simulink model "SecRwLtStLgrstInwdOtwdTrgtPosSelc"  (R2018b)
settings: Solver=FixedStepDiscrete  StartTime=0.0  StopTime=10.0  FixedStep=0.01  RelTol=1e-3
undefined symbols (not defined in the file or in its folder): KeSMSw4SAcsMd22SecRwLtStLegrstOtwdInwdPos_Val, KeSMSw4SAcsMd22SecRwLtStLegrstOtwdInwdPosMax_Val, KeSMSw4SAcsMd22SecRwLtStLegrstOtwdInwdPosMin_Val, KeSMSw4SAcsMd26SecRwLtStLegrstOtwdInwdPos_Val, KeSMSw4SAcsMd26SecRwLtStLegrstOtwdInwdPosMax_Val, KeSMSw4SAcsMd26SecRwLtStLegrstOtwdInwdPosMin_Val, KeSMSw4SLegrstCloseMdSecRwLtStLgrstOtwdInwdPos_Val, KeSMSw4SLegrstCloseMdSecRwLtStLgrstOtwdInwdPosMax_Val, KeSMSw4SLegrstCloseMdSecRwLtStLgrstOtwdInwdPosMin_Val, KeSMSw4SLegrstOpenMdSecRwLtStLgrstOtwdInwdPos_Val, KeSMSw4SLegrstOpenMdSecRwLtStLgrstOtwdInwdPosMax_Val, KeSMSw4SLegrstOpenMdSecRwLtStLgrstOtwdInwdPosMin_Val, KeSMSw4sLyingMDSecRwLtStLgrstOtwdInwdPos_160_Val, KeSMSw4sLyingMDSecRwLtStLgrstOtwdInwdPos_165_Val, KeSMSw4sLyingMDSecRwLtStLgrstOtwdInwdPos_170_Val, KeSMSw4sLyingMDSecRwLtStLgrstOtwdInwdPos_175_Val, KeSMSw4sLyingMDSecRwLtStLgrstOtwdInwdPos_180_Val, KeSMSw4sLyingMDSecRwLtStLgrstOtwdInwdPos_Below160_Val, KeSMSw4sLyingMDSecRwLtStLgrstOtwdInwdPos_Over180_Val, KeSMSw4sLyingMDSecRwLtStLgrstOtwdInwdPosMax_160_Val, KeSMSw4sLyingMDSecRwLtStLgrstOtwdInwdPosMax_165_Val, KeSMSw4sLyingMDSecRwLtStLgrstOtwdInwdPosMax_170_Val, KeSMSw4sLyingMDSecRwLtStLgrstOtwdInwdPosMax_175_Val, KeSMSw4sLyingMDSecRwLtStLgrstOtwdInwdPosMax_180_Val, KeSMSw4sLyingMDSecRwLtStLgrstOtwdInwdPosMax_Below160_Val, KeSMSw4sLyingMDSecRwLtStLgrstOtwdInwdPosMax_Over180_Val, KeSMSw4sLyingMDSecRwLtStLgrstOtwdInwdPosMin_160_Val, KeSMSw4sLyingMDSecRwLtStLgrstOtwdInwdPosMin_165_Val, KeSMSw4sLyingMDSecRwLtStLgrstOtwdInwdPosMin_170_Val, KeSMSw4sLyingMDSecRwLtStLgrstOtwdInwdPosMin_175_Val, KeSMSw4sLyingMDSecRwLtStLgrstOtwdInwdPosMin_180_Val, KeSMSw4sLyingMDSecRwLtStLgrstOtwdInwdPosMin_Below160_Val, KeSMSw4sLyingMDSecRwLtStLgrstOtwdInwdPosMin_Over180_Val, KeSMSw4sRecoveryMDSecRwLtStLgrstOtwdInwdPos_160_Val, KeSMSw4sRecoveryMDSecRwLtStLgrstOtwdInwdPos_165_Val, KeSMSw4sRecoveryMDSecRwLtStLgrstOtwdInwdPos_170_Val, KeSMSw4sRecoveryMDSecRwLtStLgrstOtwdInwdPos_175_Val, KeSMSw4sRecoveryMDSecRwLtStLgrstOtwdInwdPos_180_Val, KeSMSw4sRecoveryMDSecRwLtStLgrstOtwdInwdPos_Below160_Val, KeSMSw4sRecoveryMDSecRwLtStLgrstOtwdInwdPos_Over180_Val, KeSMSw4sRecoveryMDSecRwLtStLgrstOtwdInwdPosMax_160_Val, KeSMSw4sRecoveryMDSecRwLtStLgrstOtwdInwdPosMax_165_Val, KeSMSw4sRecoveryMDSecRwLtStLgrstOtwdInwdPosMax_170_Val, KeSMSw4sRecoveryMDSecRwLtStLgrstOtwdInwdPosMax_175_Val, KeSMSw4sRecoveryMDSecRwLtStLgrstOtwdInwdPosMax_180_Val, KeSMSw4sRecoveryMDSecRwLtStLgrstOtwdInwdPosMax_Below160_Val, KeSMSw4sRecoveryMDSecRwLtStLgrstOtwdInwdPosMax_Over180_Val, KeSMSw4sRecoveryMDSecRwLtStLgrstOtwdInwdPosMin_160_Val, KeSMSw4sRecoveryMDSecRwLtStLgrstOtwdInwdPosMin_165_Val, KeSMSw4sRecoveryMDSecRwLtStLgrstOtwdInwdPosMin_170_Val, KeSMSw4sRecoveryMDSecRwLtStLgrstOtwdInwdPosMin_175_Val, KeSMSw4sRecoveryMDSecRwLtStLgrstOtwdInwdPosMin_180_Val, KeSMSw4sRecoveryMDSecRwLtStLgrstOtwdInwdPosMin_Below160_Val, KeSMSw4sRecoveryMDSecRwLtStLgrstOtwdInwdPosMin_Over180_Val, KeSMSw4sVIPMDSecRwLtStLgrstOtwdInwdPos_160_Val, KeSMSw4sVIPMDSecRwLtStLgrstOtwdInwdPos_165_Val, KeSMSw4sVIPMDSecRwLtStLgrstOtwdInwdPos_170_Val, KeSMSw4sVIPMDSecRwLtStLgrstOtwdInwdPos_175_Val, KeSMSw4sVIPMDSecRwLtStLgrstOtwdInwdPos_180_Val, KeSMSw4sVIPMDSecRwLtStLgrstOtwdInwdPos_Below160_Val ... (+36)
libraries: TrgtPosSelcLib x12
(part 1 of 2)
settings Model: Creator=sn2xws  LastModifiedBy=sn2xws
settings Model: ModifiedHistory=|
  | 2023.8.1 V2.0.0 CR401790 增加模式21-26
  | 2024.5.6 V3.0.0 557 67座增加腿托延伸
  | 2024.7.8 V3.0.1 557模式流程V1.9
settings DataIOCC: SaveFormat=StructureWithTime
settings OptimizationCC: DefaultParameterBehavior=Inlined  EnhancedBackFolding=on  PassReuseOutputArgsAs=Individual arguments  ZeroExternalMemoryAtStartup=off  ZeroInternalMemoryAtStartup=off  OptimizeBlockOrder=speed  DifferentSizesBufferReuse=on  OptimizationCustomize=off
settings DebuggingCC: ParameterTunabilityLossMsg=error
settings ModelReferenceCC: ModelReferenceNumInstancesAllowed=Single
settings SFSimCC: MATLABDynamicMemAlloc=off
settings RTWCC: SystemTargetFile=autosar.tlc  GenCodeOnly=on  TemplateMakefile=ert_default_tmf  Description=AUTOSAR  GenerateReport=on  IncludeHyperlinkInReport=on  LaunchReport=on  GenerateTraceInfo=on  GenerateTraceReport=on  GenerateTraceReportSl=on  GenerateTraceReportSf=on  GenerateTraceReportEml=on  GenerateCodeMetricsReport=on
settings CodeAppCC: ForceParamTrailComments=on  IgnoreCustomStorageClasses=off  OperatorAnnotations=on  SimulinkDataObjDesc=on  SFDataObjDesc=on  InsertBlockDesc=on
settings STFCustomTargetCC: TargetLangStandard=C99 (ISO)  MultiwordLength=256  ParMdlRefBuildCompliant=on  CompOptLevelCompliant=on  IncludeMdlTerminateFcn=off  CombineOutputUpdateFcns=on  SuppressErrorStatus=on  ERTCustomFileBanners=on  SupportNonFinite=off  SupportComplex=off  SupportContinuousTime=off  SupportNonInlinedSFcns=off  RemoveResetFunc=on  MATLABClassNameForMDSCustomization=Simulink.SoftwareTarget.ERTCustomization  AutosarCompliant=on  UseToolchainInfoCompliant=on  LookupTableObjectStructAxisOrder=2,1,3,4,...  LUTObjectStructOrderEvenSpacing=Size,Table,Breakpoints  SystemTargetFile=autosar.tlc
settings ERTTargetCC: TargetLangStandard=C99 (ISO)  ConcurrentExecutionCompliant=off  IncludeMdlTerminateFcn=off  SuppressErrorStatus=on  SupportNonFinite=off  SupportComplex=off  ModelStepFunctionPrototypeControlCompliant=off  CPPClassGenCompliant=off  AutosarCompliant=on  LookupTableObjectStructAxisOrder=2,1,3,4,...  LUTObjectStructOrderEvenSpacing=Size,Table,Breakpoints  InlinedParameterPlacement=NonHierarchical  ERTCustomFileTemplate=example_file_process.tlc  ERTFilePackagingFormat=Compact

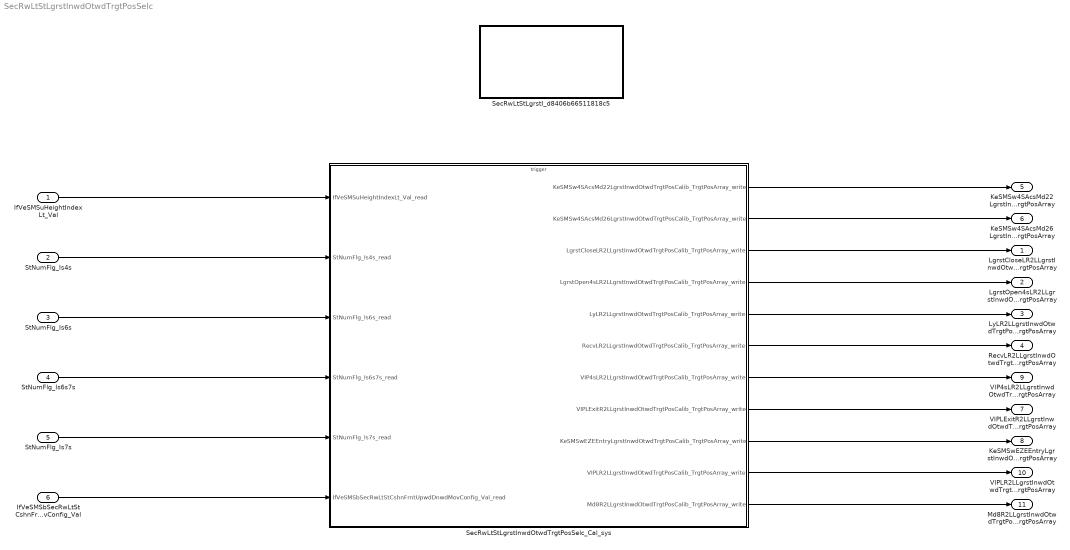
== system SecRwLtStLgrstInwdOtwdTrgtPosSelc ==
  IfVeSMSuHeightIndexLt_Val : Inport  Description=|  OutDataTypeStr=uint8  PortDimensions=1
      | 0：under 160
      | 1：160
      | 2：165
      | 3：170
      | 4：175
      | 5：180
      | 6：over 180
  StNumFlg_Is4s : Inport  Port=2  OutDataTypeStr=boolean  PortDimensions=1
  StNumFlg_Is6s : Inport  Port=3  OutDataTypeStr=boolean  PortDimensions=1
  StNumFlg_Is6s7s : Inport  Port=4  OutDataTypeStr=boolean  PortDimensions=1
  StNumFlg_Is7s : Inport  Port=5  OutDataTypeStr=boolean  PortDimensions=1
  IfVeSMSbSecRwLtStCshnFrntUpwdDnwdMovConfig_Val : Inport  Port=6  OutDataTypeStr=boolean  PortDimensions=1
  SecRwLtStLgrstI_d8406b66511818c5 : Subsystem
  SecRwLtStLgrstInwdOtwdTrgtPosSelc_Cal_sys : Subsystem
  LgrstCloseLR2LLgrstInwdOtwdTrgtPosCalib_TrgtPosArray : Outport  Description=|  OutDataTypeStr=uint16  PortDimensions=3
      | 0:Pos
      | 1:Max
      | 2:Min
  LgrstOpen4sLR2LLgrstInwdOtwdTrgtPosCalib_TrgtPosArray : Outport  Description=|  Port=2  OutDataTypeStr=uint16  PortDimensions=3
      | 0:Pos
      | 1:Max
      | 2:Min
  LyLR2LLgrstInwdOtwdTrgtPosCalib_TrgtPosArray : Outport  Description=|  Port=3  OutDataTypeStr=uint16  PortDimensions=3
      | 0:Pos
      | 1:Max
      | 2:Min
  RecvLR2LLgrstInwdOtwdTrgtPosCalib_TrgtPosArray : Outport  Description=|  Port=4  OutDataTypeStr=uint16  PortDimensions=3
      | 0:Pos
      | 1:Max
      | 2:Min
  KeSMSw4SAcsMd22LgrstInwdOtwdTrgtPosCalib_TrgtPosArray : Outport  Description=|  Port=5  OutDataTypeStr=uint16  PortDimensions=3
      | 0:Pos
      | 1:Max
      | 2:Min
  KeSMSw4SAcsMd26LgrstInwdOtwdTrgtPosCalib_TrgtPosArray : Outport  Description=|  Port=6  OutDataTypeStr=uint16  PortDimensions=3
      | 0:Pos
      | 1:Max
      | 2:Min
  VIPLExitR2LLgrstInwdOtwdTrgtPosCalib_TrgtPosArray : Outport  Description=|  Port=7  OutDataTypeStr=uint16  PortDimensions=3
      | 0:Pos
      | 1:Max
      | 2:Min
  KeSMSwEZEEntryLgrstInwdOtwdTrgtPosCalib_TrgtPosArray : Outport  Description=|  Port=8  OutDataTypeStr=uint16  PortDimensions=3
      | 0:Pos
      | 1:Max
      | 2:Min
  VIP4sLR2LLgrstInwdOtwdTrgtPosCalib_TrgtPosArray : Outport  Description=|  Port=9  OutDataTypeStr=uint16  PortDimensions=3
      | 0:Pos
      | 1:Max
      | 2:Min
  VIPLR2LLgrstInwdOtwdTrgtPosCalib_TrgtPosArray : Outport  Description=|  Port=10  OutDataTypeStr=uint16  PortDimensions=3
      | 0:Pos
      | 1:Max
      | 2:Min
  Md8R2LLgrstInwdOtwdTrgtPosCalib_TrgtPosArray : Outport  Description=|  Port=11  OutDataTypeStr=uint16  PortDimensions=3
      | 0:Pos
      | 1:Max
      | 2:Min
  wires:
  IfVeSMSuHeightIndexLt_Val/1 -> SecRwLtStLgrstInwdOtwdTrgtPosSelc_Cal_sys/1(IfVeSMSuHeightIndexLt_Val_read)
  StNumFlg_Is4s/1 -> SecRwLtStLgrstInwdOtwdTrgtPosSelc_Cal_sys/2(StNumFlg_Is4s_read)
  StNumFlg_Is6s/1 -> SecRwLtStLgrstInwdOtwdTrgtPosSelc_Cal_sys/3(StNumFlg_Is6s_read)
  StNumFlg_Is6s7s/1 -> SecRwLtStLgrstInwdOtwdTrgtPosSelc_Cal_sys/4(StNumFlg_Is6s7s_read)
  StNumFlg_Is7s/1 -> SecRwLtStLgrstInwdOtwdTrgtPosSelc_Cal_sys/5(StNumFlg_Is7s_read)
  SecRwLtStLgrstInwdOtwdTrgtPosSelc_Cal_sys/3(LgrstCloseLR2LLgrstInwdOtwdTrgtPosCalib_TrgtPosArray_write) -> LgrstCloseLR2LLgrstInwdOtwdTrgtPosCalib_TrgtPosArray/1
  SecRwLtStLgrstInwdOtwdTrgtPosSelc_Cal_sys/4(LgrstOpen4sLR2LLgrstInwdOtwdTrgtPosCalib_TrgtPosArray_write) -> LgrstOpen4sLR2LLgrstInwdOtwdTrgtPosCalib_TrgtPosArray/1
  SecRwLtStLgrstInwdOtwdTrgtPosSelc_Cal_sys/5(LyLR2LLgrstInwdOtwdTrgtPosCalib_TrgtPosArray_write) -> LyLR2LLgrstInwdOtwdTrgtPosCalib_TrgtPosArray/1
  SecRwLtStLgrstInwdOtwdTrgtPosSelc_Cal_sys/6(RecvLR2LLgrstInwdOtwdTrgtPosCalib_TrgtPosArray_write) -> RecvLR2LLgrstInwdOtwdTrgtPosCalib_TrgtPosArray/1
  SecRwLtStLgrstInwdOtwdTrgtPosSelc_Cal_sys/1(KeSMSw4SAcsMd22LgrstInwdOtwdTrgtPosCalib_TrgtPosArray_write) -> KeSMSw4SAcsMd22LgrstInwdOtwdTrgtPosCalib_TrgtPosArray/1
  SecRwLtStLgrstInwdOtwdTrgtPosSelc_Cal_sys/2(KeSMSw4SAcsMd26LgrstInwdOtwdTrgtPosCalib_TrgtPosArray_write) -> KeSMSw4SAcsMd26LgrstInwdOtwdTrgtPosCalib_TrgtPosArray/1
  IfVeSMSbSecRwLtStCshnFrntUpwdDnwdMovConfig_Val/1 -> SecRwLtStLgrstInwdOtwdTrgtPosSelc_Cal_sys/6(IfVeSMSbSecRwLtStCshnFrntUpwdDnwdMovConfig_Val_read)
  SecRwLtStLgrstInwdOtwdTrgtPosSelc_Cal_sys/8(VIPLExitR2LLgrstInwdOtwdTrgtPosCalib_TrgtPosArray_write) -> VIPLExitR2LLgrstInwdOtwdTrgtPosCalib_TrgtPosArray/1
  SecRwLtStLgrstInwdOtwdTrgtPosSelc_Cal_sys/9(KeSMSwEZEEntryLgrstInwdOtwdTrgtPosCalib_TrgtPosArray_write) -> KeSMSwEZEEntryLgrstInwdOtwdTrgtPosCalib_TrgtPosArray/1
  SecRwLtStLgrstInwdOtwdTrgtPosSelc_Cal_sys/7(VIP4sLR2LLgrstInwdOtwdTrgtPosCalib_TrgtPosArray_write) -> VIP4sLR2LLgrstInwdOtwdTrgtPosCalib_TrgtPosArray/1
  SecRwLtStLgrstInwdOtwdTrgtPosSelc_Cal_sys/10(VIPLR2LLgrstInwdOtwdTrgtPosCalib_TrgtPosArray_write) -> VIPLR2LLgrstInwdOtwdTrgtPosCalib_TrgtPosArray/1
  SecRwLtStLgrstInwdOtwdTrgtPosSelc_Cal_sys/11(Md8R2LLgrstInwdOtwdTrgtPosCalib_TrgtPosArray_write) -> Md8R2LLgrstInwdOtwdTrgtPosCalib_TrgtPosArray/1

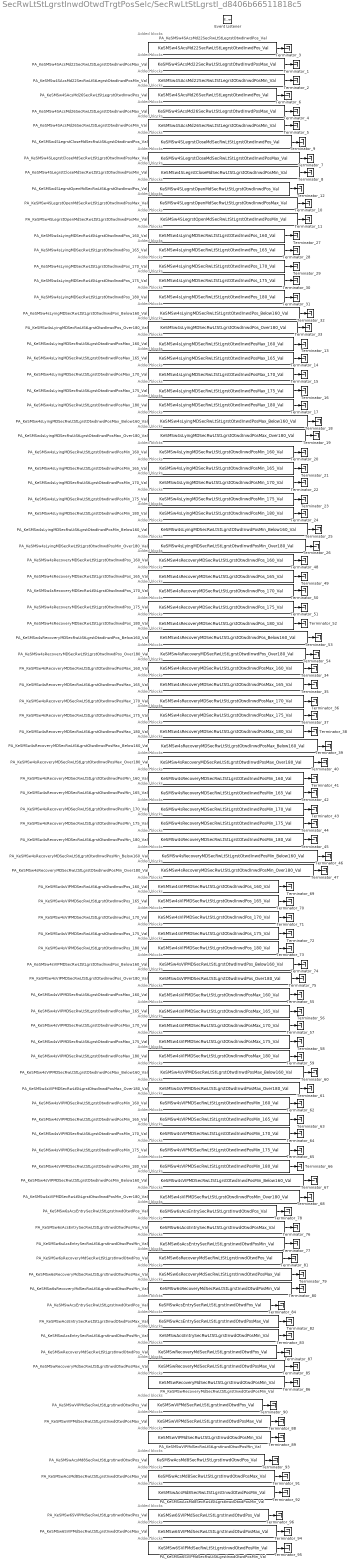
== system SecRwLtStLgrstInwdOtwdTrgtPosSelc/SecRwLtStLgrstI_d8406b66511818c5 ==
  note: Added blocks
  note: Added blocks
  note: Added blocks
  note: Added blocks
  note: Added blocks
  note: Added blocks
  note: Added blocks
  note: Added blocks
  note: Added blocks
  note: Added blocks
  note: Added blocks
  note: Added blocks
  note: Added blocks
  note: Added blocks
  note: Added blocks
  note: Added blocks
  note: Added blocks
  note: Added blocks
  note: Added blocks
  note: Added blocks
  note: Added blocks
  note: Added blocks
  note: Added blocks
  note: Added blocks
  note: Added blocks
  note: Added blocks
  note: Added blocks
  note: Added blocks
  note: Added blocks
  note: Added blocks
  note: Added blocks
  note: Added blocks
  note: Added blocks
  note: Added blocks
  note: Added blocks
  note: Added blocks
  note: Added blocks
  note: Added blocks
  note: Added blocks
  note: Added blocks
  note: Added blocks
  note: Added blocks
  note: Added blocks
  note: Added blocks
  note: Added blocks
  note: Added blocks
  note: Added blocks
  note: Added blocks
  note: Added blocks
  note: Added blocks
  note: Added blocks
  note: Added blocks
  note: Added blocks
  note: Added blocks
  note: Added blocks
  note: Added blocks
  note: Added blocks
  note: Added blocks
  note: Added blocks
  note: Added blocks
  note: Added blocks
  note: Added blocks
  note: Added blocks
  note: Added blocks
  note: Added blocks
  note: Added blocks
  note: Added blocks
  note: Added blocks
  note: Added blocks
  note: Added blocks
  note: Added blocks
  note: Added blocks
  note: Added blocks
  note: Added blocks
  note: Added blocks
  note: Added blocks
  note: Added blocks
  note: Added blocks
  note: Added blocks
  note: Added blocks
  note: Added blocks
  note: Added blocks
  note: Added blocks
  note: Added blocks
  note: Added blocks
  note: Added blocks
  note: Added blocks
  note: Added blocks
  note: Added blocks
  note: Added blocks
  note: Added blocks
  note: Added blocks
  note: Added blocks
  note: Added blocks
  note: Added blocks
  note: Added blocks
  Event Listener : EventListener  EventName=reset
  PA_KeSMSw4SAcsMd22SecRwLtStLegrstOtwdInwdPosMax_Val : Constant  Value=KeSMSw4SAcsMd22SecRwLtStLegrstOtwdInwdPosMax_Val
  PA_KeSMSw4SAcsMd22SecRwLtStLegrstOtwdInwdPosMin_Val : Constant  Value=KeSMSw4SAcsMd22SecRwLtStLegrstOtwdInwdPosMin_Val
  PA_KeSMSw4SAcsMd22SecRwLtStLegrstOtwdInwdPos_Val : Constant  Value=KeSMSw4SAcsMd22SecRwLtStLegrstOtwdInwdPos_Val
  PA_KeSMSw4SAcsMd26SecRwLtStLegrstOtwdInwdPosMax_Val : Constant  Value=KeSMSw4SAcsMd26SecRwLtStLegrstOtwdInwdPosMax_Val
  PA_KeSMSw4SAcsMd26SecRwLtStLegrstOtwdInwdPosMin_Val : Constant  Value=KeSMSw4SAcsMd26SecRwLtStLegrstOtwdInwdPosMin_Val
  PA_KeSMSw4SAcsMd26SecRwLtStLegrstOtwdInwdPos_Val : Constant  Value=KeSMSw4SAcsMd26SecRwLtStLegrstOtwdInwdPos_Val
  PA_KeSMSw4SLegrstCloseMdSecRwLtStLgrstOtwdInwdPosMax_Val : Constant  Value=KeSMSw4SLegrstCloseMdSecRwLtStLgrstOtwdInwdPosMax_Val
  PA_KeSMSw4SLegrstCloseMdSecRwLtStLgrstOtwdInwdPosMin_Val : Constant  Value=KeSMSw4SLegrstCloseMdSecRwLtStLgrstOtwdInwdPosMin_Val
  PA_KeSMSw4SLegrstCloseMdSecRwLtStLgrstOtwdInwdPos_Val : Constant  Value=KeSMSw4SLegrstCloseMdSecRwLtStLgrstOtwdInwdPos_Val
  PA_KeSMSw4SLegrstOpenMdSecRwLtStLgrstOtwdInwdPosMax_Val : Constant  Value=KeSMSw4SLegrstOpenMdSecRwLtStLgrstOtwdInwdPosMax_Val
  PA_KeSMSw4SLegrstOpenMdSecRwLtStLgrstOtwdInwdPosMin_Val : Constant  Value=KeSMSw4SLegrstOpenMdSecRwLtStLgrstOtwdInwdPosMin_Val
  PA_KeSMSw4SLegrstOpenMdSecRwLtStLgrstOtwdInwdPos_Val : Constant  Value=KeSMSw4SLegrstOpenMdSecRwLtStLgrstOtwdInwdPos_Val
  PA_KeSMSw4sLyingMDSecRwLtStLgrstOtwdInwdPosMax_160_Val : Constant  Value=KeSMSw4sLyingMDSecRwLtStLgrstOtwdInwdPosMax_160_Val
  PA_KeSMSw4sLyingMDSecRwLtStLgrstOtwdInwdPosMax_165_Val : Constant  Value=KeSMSw4sLyingMDSecRwLtStLgrstOtwdInwdPosMax_165_Val
  PA_KeSMSw4sLyingMDSecRwLtStLgrstOtwdInwdPosMax_170_Val : Constant  Value=KeSMSw4sLyingMDSecRwLtStLgrstOtwdInwdPosMax_170_Val
  PA_KeSMSw4sLyingMDSecRwLtStLgrstOtwdInwdPosMax_175_Val : Constant  Value=KeSMSw4sLyingMDSecRwLtStLgrstOtwdInwdPosMax_175_Val
  PA_KeSMSw4sLyingMDSecRwLtStLgrstOtwdInwdPosMax_180_Val : Constant  Value=KeSMSw4sLyingMDSecRwLtStLgrstOtwdInwdPosMax_180_Val
  PA_KeSMSw4sLyingMDSecRwLtStLgrstOtwdInwdPosMax_Below160_Val : Constant  Value=KeSMSw4sLyingMDSecRwLtStLgrstOtwdInwdPosMax_Below160_Val
  PA_KeSMSw4sLyingMDSecRwLtStLgrstOtwdInwdPosMax_Over180_Val : Constant  Value=KeSMSw4sLyingMDSecRwLtStLgrstOtwdInwdPosMax_Over180_Val
  PA_KeSMSw4sLyingMDSecRwLtStLgrstOtwdInwdPosMin_160_Val : Constant  Value=KeSMSw4sLyingMDSecRwLtStLgrstOtwdInwdPosMin_160_Val
  PA_KeSMSw4sLyingMDSecRwLtStLgrstOtwdInwdPosMin_165_Val : Constant  Value=KeSMSw4sLyingMDSecRwLtStLgrstOtwdInwdPosMin_165_Val
  PA_KeSMSw4sLyingMDSecRwLtStLgrstOtwdInwdPosMin_170_Val : Constant  Value=KeSMSw4sLyingMDSecRwLtStLgrstOtwdInwdPosMin_170_Val
  PA_KeSMSw4sLyingMDSecRwLtStLgrstOtwdInwdPosMin_175_Val : Constant  Value=KeSMSw4sLyingMDSecRwLtStLgrstOtwdInwdPosMin_175_Val
  PA_KeSMSw4sLyingMDSecRwLtStLgrstOtwdInwdPosMin_180_Val : Constant  Value=KeSMSw4sLyingMDSecRwLtStLgrstOtwdInwdPosMin_180_Val
  PA_KeSMSw4sLyingMDSecRwLtStLgrstOtwdInwdPosMin_Below160_Val : Constant  Value=KeSMSw4sLyingMDSecRwLtStLgrstOtwdInwdPosMin_Below160_Val
  PA_KeSMSw4sLyingMDSecRwLtStLgrstOtwdInwdPosMin_Over180_Val : Constant  Value=KeSMSw4sLyingMDSecRwLtStLgrstOtwdInwdPosMin_Over180_Val
  PA_KeSMSw4sLyingMDSecRwLtStLgrstOtwdInwdPos_160_Val : Constant  Value=KeSMSw4sLyingMDSecRwLtStLgrstOtwdInwdPos_160_Val
  PA_KeSMSw4sLyingMDSecRwLtStLgrstOtwdInwdPos_165_Val : Constant  Value=KeSMSw4sLyingMDSecRwLtStLgrstOtwdInwdPos_165_Val
  PA_KeSMSw4sLyingMDSecRwLtStLgrstOtwdInwdPos_170_Val : Constant  Value=KeSMSw4sLyingMDSecRwLtStLgrstOtwdInwdPos_170_Val
  PA_KeSMSw4sLyingMDSecRwLtStLgrstOtwdInwdPos_175_Val : Constant  Value=KeSMSw4sLyingMDSecRwLtStLgrstOtwdInwdPos_175_Val
  PA_KeSMSw4sLyingMDSecRwLtStLgrstOtwdInwdPos_180_Val : Constant  Value=KeSMSw4sLyingMDSecRwLtStLgrstOtwdInwdPos_180_Val
  PA_KeSMSw4sLyingMDSecRwLtStLgrstOtwdInwdPos_Below160_Val : Constant  Value=KeSMSw4sLyingMDSecRwLtStLgrstOtwdInwdPos_Below160_Val
  PA_KeSMSw4sLyingMDSecRwLtStLgrstOtwdInwdPos_Over180_Val : Constant  Value=KeSMSw4sLyingMDSecRwLtStLgrstOtwdInwdPos_Over180_Val
  PA_KeSMSw4sRecoveryMDSecRwLtStLgrstOtwdInwdPosMax_160_Val : Constant  Value=KeSMSw4sRecoveryMDSecRwLtStLgrstOtwdInwdPosMax_160_Val
  PA_KeSMSw4sRecoveryMDSecRwLtStLgrstOtwdInwdPosMax_165_Val : Constant  Value=KeSMSw4sRecoveryMDSecRwLtStLgrstOtwdInwdPosMax_165_Val
  PA_KeSMSw4sRecoveryMDSecRwLtStLgrstOtwdInwdPosMax_170_Val : Constant  Value=KeSMSw4sRecoveryMDSecRwLtStLgrstOtwdInwdPosMax_170_Val
  PA_KeSMSw4sRecoveryMDSecRwLtStLgrstOtwdInwdPosMax_175_Val : Constant  Value=KeSMSw4sRecoveryMDSecRwLtStLgrstOtwdInwdPosMax_175_Val
  PA_KeSMSw4sRecoveryMDSecRwLtStLgrstOtwdInwdPosMax_180_Val : Constant  Value=KeSMSw4sRecoveryMDSecRwLtStLgrstOtwdInwdPosMax_180_Val
  PA_KeSMSw4sRecoveryMDSecRwLtStLgrstOtwdInwdPosMax_Below160_Val : Constant  Value=KeSMSw4sRecoveryMDSecRwLtStLgrstOtwdInwdPosMax_Below160_Val
  PA_KeSMSw4sRecoveryMDSecRwLtStLgrstOtwdInwdPosMax_Over180_Val : Constant  Value=KeSMSw4sRecoveryMDSecRwLtStLgrstOtwdInwdPosMax_Over180_Val
  PA_KeSMSw4sRecoveryMDSecRwLtStLgrstOtwdInwdPosMin_160_Val : Constant  Value=KeSMSw4sRecoveryMDSecRwLtStLgrstOtwdInwdPosMin_160_Val
  PA_KeSMSw4sRecoveryMDSecRwLtStLgrstOtwdInwdPosMin_165_Val : Constant  Value=KeSMSw4sRecoveryMDSecRwLtStLgrstOtwdInwdPosMin_165_Val
  PA_KeSMSw4sRecoveryMDSecRwLtStLgrstOtwdInwdPosMin_170_Val : Constant  Value=KeSMSw4sRecoveryMDSecRwLtStLgrstOtwdInwdPosMin_170_Val
  PA_KeSMSw4sRecoveryMDSecRwLtStLgrstOtwdInwdPosMin_175_Val : Constant  Value=KeSMSw4sRecoveryMDSecRwLtStLgrstOtwdInwdPosMin_175_Val
  PA_KeSMSw4sRecoveryMDSecRwLtStLgrstOtwdInwdPosMin_180_Val : Constant  Value=KeSMSw4sRecoveryMDSecRwLtStLgrstOtwdInwdPosMin_180_Val
  PA_KeSMSw4sRecoveryMDSecRwLtStLgrstOtwdInwdPosMin_Below160_Val : Constant  Value=KeSMSw4sRecoveryMDSecRwLtStLgrstOtwdInwdPosMin_Below160_Val
  PA_KeSMSw4sRecoveryMDSecRwLtStLgrstOtwdInwdPosMin_Over180_Val : Constant  Value=KeSMSw4sRecoveryMDSecRwLtStLgrstOtwdInwdPosMin_Over180_Val
  PA_KeSMSw4sRecoveryMDSecRwLtStLgrstOtwdInwdPos_160_Val : Constant  Value=KeSMSw4sRecoveryMDSecRwLtStLgrstOtwdInwdPos_160_Val
  PA_KeSMSw4sRecoveryMDSecRwLtStLgrstOtwdInwdPos_165_Val : Constant  Value=KeSMSw4sRecoveryMDSecRwLtStLgrstOtwdInwdPos_165_Val
  PA_KeSMSw4sRecoveryMDSecRwLtStLgrstOtwdInwdPos_170_Val : Constant  Value=KeSMSw4sRecoveryMDSecRwLtStLgrstOtwdInwdPos_170_Val
  PA_KeSMSw4sRecoveryMDSecRwLtStLgrstOtwdInwdPos_175_Val : Constant  Value=KeSMSw4sRecoveryMDSecRwLtStLgrstOtwdInwdPos_175_Val
  PA_KeSMSw4sRecoveryMDSecRwLtStLgrstOtwdInwdPos_180_Val : Constant  Value=KeSMSw4sRecoveryMDSecRwLtStLgrstOtwdInwdPos_180_Val
  PA_KeSMSw4sRecoveryMDSecRwLtStLgrstOtwdInwdPos_Below160_Val : Constant  Value=KeSMSw4sRecoveryMDSecRwLtStLgrstOtwdInwdPos_Below160_Val
  PA_KeSMSw4sRecoveryMDSecRwLtStLgrstOtwdInwdPos_Over180_Val : Constant  Value=KeSMSw4sRecoveryMDSecRwLtStLgrstOtwdInwdPos_Over180_Val
  PA_KeSMSw4sVIPMDSecRwLtStLgrstOtwdInwdPosMax_160_Val : Constant  Value=KeSMSw4sVIPMDSecRwLtStLgrstOtwdInwdPosMax_160_Val
  PA_KeSMSw4sVIPMDSecRwLtStLgrstOtwdInwdPosMax_165_Val : Constant  Value=KeSMSw4sVIPMDSecRwLtStLgrstOtwdInwdPosMax_165_Val
  PA_KeSMSw4sVIPMDSecRwLtStLgrstOtwdInwdPosMax_170_Val : Constant  Value=KeSMSw4sVIPMDSecRwLtStLgrstOtwdInwdPosMax_170_Val
  PA_KeSMSw4sVIPMDSecRwLtStLgrstOtwdInwdPosMax_175_Val : Constant  Value=KeSMSw4sVIPMDSecRwLtStLgrstOtwdInwdPosMax_175_Val
  PA_KeSMSw4sVIPMDSecRwLtStLgrstOtwdInwdPosMax_180_Val : Constant  Value=KeSMSw4sVIPMDSecRwLtStLgrstOtwdInwdPosMax_180_Val
  PA_KeSMSw4sVIPMDSecRwLtStLgrstOtwdInwdPosMax_Below160_Val : Constant  Value=KeSMSw4sVIPMDSecRwLtStLgrstOtwdInwdPosMax_Below160_Val
  PA_KeSMSw4sVIPMDSecRwLtStLgrstOtwdInwdPosMax_Over180_Val : Constant  Value=KeSMSw4sVIPMDSecRwLtStLgrstOtwdInwdPosMax_Over180_Val
  PA_KeSMSw4sVIPMDSecRwLtStLgrstOtwdInwdPosMin_160_Val : Constant  Value=KeSMSw4sVIPMDSecRwLtStLgrstOtwdInwdPosMin_160_Val
  PA_KeSMSw4sVIPMDSecRwLtStLgrstOtwdInwdPosMin_165_Val : Constant  Value=KeSMSw4sVIPMDSecRwLtStLgrstOtwdInwdPosMin_165_Val
  PA_KeSMSw4sVIPMDSecRwLtStLgrstOtwdInwdPosMin_170_Val : Constant  Value=KeSMSw4sVIPMDSecRwLtStLgrstOtwdInwdPosMin_170_Val
  PA_KeSMSw4sVIPMDSecRwLtStLgrstOtwdInwdPosMin_175_Val : Constant  Value=KeSMSw4sVIPMDSecRwLtStLgrstOtwdInwdPosMin_175_Val
  PA_KeSMSw4sVIPMDSecRwLtStLgrstOtwdInwdPosMin_180_Val : Constant  Value=KeSMSw4sVIPMDSecRwLtStLgrstOtwdInwdPosMin_180_Val
  PA_KeSMSw4sVIPMDSecRwLtStLgrstOtwdInwdPosMin_Below160_Val : Constant  Value=KeSMSw4sVIPMDSecRwLtStLgrstOtwdInwdPosMin_Below160_Val
  PA_KeSMSw4sVIPMDSecRwLtStLgrstOtwdInwdPosMin_Over180_Val : Constant  Value=KeSMSw4sVIPMDSecRwLtStLgrstOtwdInwdPosMin_Over180_Val
  PA_KeSMSw4sVIPMDSecRwLtStLgrstOtwdInwdPos_160_Val : Constant  Value=KeSMSw4sVIPMDSecRwLtStLgrstOtwdInwdPos_160_Val
  PA_KeSMSw4sVIPMDSecRwLtStLgrstOtwdInwdPos_165_Val : Constant  Value=KeSMSw4sVIPMDSecRwLtStLgrstOtwdInwdPos_165_Val
  PA_KeSMSw4sVIPMDSecRwLtStLgrstOtwdInwdPos_170_Val : Constant  Value=KeSMSw4sVIPMDSecRwLtStLgrstOtwdInwdPos_170_Val
  PA_KeSMSw4sVIPMDSecRwLtStLgrstOtwdInwdPos_175_Val : Constant  Value=KeSMSw4sVIPMDSecRwLtStLgrstOtwdInwdPos_175_Val
  PA_KeSMSw4sVIPMDSecRwLtStLgrstOtwdInwdPos_180_Val : Constant  Value=KeSMSw4sVIPMDSecRwLtStLgrstOtwdInwdPos_180_Val
  PA_KeSMSw4sVIPMDSecRwLtStLgrstOtwdInwdPos_Below160_Val : Constant  Value=KeSMSw4sVIPMDSecRwLtStLgrstOtwdInwdPos_Below160_Val
  PA_KeSMSw4sVIPMDSecRwLtStLgrstOtwdInwdPos_Over180_Val : Constant  Value=KeSMSw4sVIPMDSecRwLtStLgrstOtwdInwdPos_Over180_Val
  PA_KeSMSw6SVIPMdSecRwLtStLgrstInwdOtwdPosMax_Val : Constant  Value=KeSMSw6SVIPMdSecRwLtStLgrstInwdOtwdPosMax_Val
  PA_KeSMSw6SVIPMdSecRwLtStLgrstInwdOtwdPosMin_Val : Constant  Value=KeSMSw6SVIPMdSecRwLtStLgrstInwdOtwdPosMin_Val
  PA_KeSMSw6SVIPMdSecRwLtStLgrstInwdOtwdPos_Val : Constant  Value=KeSMSw6SVIPMdSecRwLtStLgrstInwdOtwdPos_Val
  PA_KeSMSw6sAcsEntrySecRwLtStLgrstInwdOtwdPosMax_Val : Constant  Value=KeSMSw6sAcsEntrySecRwLtStLgrstInwdOtwdPosMax_Val
  PA_KeSMSw6sAcsEntrySecRwLtStLgrstInwdOtwdPosMin_Val : Constant  Value=KeSMSw6sAcsEntrySecRwLtStLgrstInwdOtwdPosMin_Val
  PA_KeSMSw6sAcsEntrySecRwLtStLgrstInwdOtwdPos_Val : Constant  Value=KeSMSw6sAcsEntrySecRwLtStLgrstInwdOtwdPos_Val
  PA_KeSMSw6sRecoveryMdSecRwLtStLgrstInwdOtwdPosMax_Val : Constant  Value=KeSMSw6sRecoveryMdSecRwLtStLgrstInwdOtwdPosMax_Val
  PA_KeSMSw6sRecoveryMdSecRwLtStLgrstInwdOtwdPosMin_Val : Constant  Value=KeSMSw6sRecoveryMdSecRwLtStLgrstInwdOtwdPosMin_Val
  PA_KeSMSw6sRecoveryMdSecRwLtStLgrstInwdOtwdPos_Val : Constant  Value=KeSMSw6sRecoveryMdSecRwLtStLgrstInwdOtwdPos_Val
  PA_KeSMSwAcsEntrySecRwLtStLgrstInwdOtwdPosMax_Val : Constant  Value=KeSMSwAcsEntrySecRwLtStLgrstInwdOtwdPosMax_Val
  PA_KeSMSwAcsEntrySecRwLtStLgrstInwdOtwdPosMin_Val : Constant  Value=KeSMSwAcsEntrySecRwLtStLgrstInwdOtwdPosMin_Val
  PA_KeSMSwAcsEntrySecRwLtStLgrstInwdOtwdPos_Val : Constant  Value=KeSMSwAcsEntrySecRwLtStLgrstInwdOtwdPos_Val
  PA_KeSMSwAcsMd8SecRwLtStLgrstInwdOtwdPosMax_Val : Constant  Value=KeSMSwAcsMd8SecRwLtStLgrstInwdOtwdPosMax_Val
  PA_KeSMSwAcsMd8SecRwLtStLgrstInwdOtwdPosMin_Val : Constant  Value=KeSMSwAcsMd8SecRwLtStLgrstInwdOtwdPosMin_Val
  PA_KeSMSwAcsMd8SecRwLtStLgrstInwdOtwdPos_Val : Constant  Value=KeSMSwAcsMd8SecRwLtStLgrstInwdOtwdPos_Val
  PA_KeSMSwRecoveryMdSecRwLtStLgrstInwdOtwdPosMax_Val : Constant  Value=KeSMSwRecoveryMdSecRwLtStLgrstInwdOtwdPosMax_Val
  PA_KeSMSwRecoveryMdSecRwLtStLgrstInwdOtwdPosMin_Val : Constant  Value=KeSMSwRecoveryMdSecRwLtStLgrstInwdOtwdPosMin_Val
  PA_KeSMSwRecoveryMdSecRwLtStLgrstInwdOtwdPos_Val : Constant  Value=KeSMSwRecoveryMdSecRwLtStLgrstInwdOtwdPos_Val
  PA_KeSMSwVIPMdSecRwLtStLgrstInwdOtwdPosMax_Val : Constant  Value=KeSMSwVIPMdSecRwLtStLgrstInwdOtwdPosMax_Val
  PA_KeSMSwVIPMdSecRwLtStLgrstInwdOtwdPosMin_Val : Constant  Value=KeSMSwVIPMdSecRwLtStLgrstInwdOtwdPosMin_Val
  PA_KeSMSwVIPMdSecRwLtStLgrstInwdOtwdPos_Val : Constant  Value=KeSMSwVIPMdSecRwLtStLgrstInwdOtwdPos_Val
  Terminator_{1..96} (96 alike) : Terminator
  wires:
  PA_KeSMSw4SAcsMd22SecRwLtStLegrstOtwdInwdPosMax_Val/1 -> Terminator_1/1
  PA_KeSMSw4SAcsMd22SecRwLtStLegrstOtwdInwdPosMin_Val/1 -> Terminator_2/1
  PA_KeSMSw4SAcsMd22SecRwLtStLegrstOtwdInwdPos_Val/1 -> Terminator_3/1
  PA_KeSMSw4SAcsMd26SecRwLtStLegrstOtwdInwdPosMax_Val/1 -> Terminator_4/1
  PA_KeSMSw4SAcsMd26SecRwLtStLegrstOtwdInwdPosMin_Val/1 -> Terminator_5/1
  PA_KeSMSw4SAcsMd26SecRwLtStLegrstOtwdInwdPos_Val/1 -> Terminator_6/1
  PA_KeSMSw4SLegrstCloseMdSecRwLtStLgrstOtwdInwdPosMax_Val/1 -> Terminator_7/1
  PA_KeSMSw4SLegrstCloseMdSecRwLtStLgrstOtwdInwdPosMin_Val/1 -> Terminator_8/1
  PA_KeSMSw4SLegrstCloseMdSecRwLtStLgrstOtwdInwdPos_Val/1 -> Terminator_9/1
  PA_KeSMSw4SLegrstOpenMdSecRwLtStLgrstOtwdInwdPosMax_Val/1 -> Terminator_10/1
  PA_KeSMSw4SLegrstOpenMdSecRwLtStLgrstOtwdInwdPosMin_Val/1 -> Terminator_11/1
  PA_KeSMSw4SLegrstOpenMdSecRwLtStLgrstOtwdInwdPos_Val/1 -> Terminator_12/1
  PA_KeSMSw4sLyingMDSecRwLtStLgrstOtwdInwdPosMax_160_Val/1 -> Terminator_13/1
  PA_KeSMSw4sLyingMDSecRwLtStLgrstOtwdInwdPosMax_165_Val/1 -> Terminator_14/1
  PA_KeSMSw4sLyingMDSecRwLtStLgrstOtwdInwdPosMax_170_Val/1 -> Terminator_15/1
  PA_KeSMSw4sLyingMDSecRwLtStLgrstOtwdInwdPosMax_175_Val/1 -> Terminator_16/1
  PA_KeSMSw4sLyingMDSecRwLtStLgrstOtwdInwdPosMax_180_Val/1 -> Terminator_17/1
  PA_KeSMSw4sLyingMDSecRwLtStLgrstOtwdInwdPosMax_Below160_Val/1 -> Terminator_18/1
  PA_KeSMSw4sLyingMDSecRwLtStLgrstOtwdInwdPosMax_Over180_Val/1 -> Terminator_19/1
  PA_KeSMSw4sLyingMDSecRwLtStLgrstOtwdInwdPosMin_160_Val/1 -> Terminator_20/1
  PA_KeSMSw4sLyingMDSecRwLtStLgrstOtwdInwdPosMin_165_Val/1 -> Terminator_21/1
  PA_KeSMSw4sLyingMDSecRwLtStLgrstOtwdInwdPosMin_170_Val/1 -> Terminator_22/1
  PA_KeSMSw4sLyingMDSecRwLtStLgrstOtwdInwdPosMin_175_Val/1 -> Terminator_23/1
  PA_KeSMSw4sLyingMDSecRwLtStLgrstOtwdInwdPosMin_180_Val/1 -> Terminator_24/1
  PA_KeSMSw4sLyingMDSecRwLtStLgrstOtwdInwdPosMin_Below160_Val/1 -> Terminator_25/1
  PA_KeSMSw4sLyingMDSecRwLtStLgrstOtwdInwdPosMin_Over180_Val/1 -> Terminator_26/1
  PA_KeSMSw4sLyingMDSecRwLtStLgrstOtwdInwdPos_160_Val/1 -> Terminator_27/1
  PA_KeSMSw4sLyingMDSecRwLtStLgrstOtwdInwdPos_165_Val/1 -> Terminator_28/1
  PA_KeSMSw4sLyingMDSecRwLtStLgrstOtwdInwdPos_170_Val/1 -> Terminator_29/1
  PA_KeSMSw4sLyingMDSecRwLtStLgrstOtwdInwdPos_175_Val/1 -> Terminator_30/1
  PA_KeSMSw4sLyingMDSecRwLtStLgrstOtwdInwdPos_180_Val/1 -> Terminator_31/1
  PA_KeSMSw4sLyingMDSecRwLtStLgrstOtwdInwdPos_Below160_Val/1 -> Terminator_32/1
  PA_KeSMSw4sLyingMDSecRwLtStLgrstOtwdInwdPos_Over180_Val/1 -> Terminator_33/1
  PA_KeSMSw4sRecoveryMDSecRwLtStLgrstOtwdInwdPosMax_160_Val/1 -> Terminator_34/1
  PA_KeSMSw4sRecoveryMDSecRwLtStLgrstOtwdInwdPosMax_165_Val/1 -> Terminator_35/1
  PA_KeSMSw4sRecoveryMDSecRwLtStLgrstOtwdInwdPosMax_170_Val/1 -> Terminator_36/1
  PA_KeSMSw4sRecoveryMDSecRwLtStLgrstOtwdInwdPosMax_175_Val/1 -> Terminator_37/1
  PA_KeSMSw4sRecoveryMDSecRwLtStLgrstOtwdInwdPosMax_180_Val/1 -> Terminator_38/1
  PA_KeSMSw4sRecoveryMDSecRwLtStLgrstOtwdInwdPosMax_Below160_Val/1 -> Terminator_39/1
  PA_KeSMSw4sRecoveryMDSecRwLtStLgrstOtwdInwdPosMax_Over180_Val/1 -> Terminator_40/1
  PA_KeSMSw4sRecoveryMDSecRwLtStLgrstOtwdInwdPosMin_160_Val/1 -> Terminator_41/1
  PA_KeSMSw4sRecoveryMDSecRwLtStLgrstOtwdInwdPosMin_165_Val/1 -> Terminator_42/1
  PA_KeSMSw4sRecoveryMDSecRwLtStLgrstOtwdInwdPosMin_170_Val/1 -> Terminator_43/1
  PA_KeSMSw4sRecoveryMDSecRwLtStLgrstOtwdInwdPosMin_175_Val/1 -> Terminator_44/1
  PA_KeSMSw4sRecoveryMDSecRwLtStLgrstOtwdInwdPosMin_180_Val/1 -> Terminator_45/1
  PA_KeSMSw4sRecoveryMDSecRwLtStLgrstOtwdInwdPosMin_Below160_Val/1 -> Terminator_46/1
  PA_KeSMSw4sRecoveryMDSecRwLtStLgrstOtwdInwdPosMin_Over180_Val/1 -> Terminator_47/1
  PA_KeSMSw4sRecoveryMDSecRwLtStLgrstOtwdInwdPos_160_Val/1 -> Terminator_48/1
  PA_KeSMSw4sRecoveryMDSecRwLtStLgrstOtwdInwdPos_165_Val/1 -> Terminator_49/1
  PA_KeSMSw4sRecoveryMDSecRwLtStLgrstOtwdInwdPos_170_Val/1 -> Terminator_50/1
  PA_KeSMSw4sRecoveryMDSecRwLtStLgrstOtwdInwdPos_175_Val/1 -> Terminator_51/1
  PA_KeSMSw4sRecoveryMDSecRwLtStLgrstOtwdInwdPos_180_Val/1 -> Terminator_52/1
  PA_KeSMSw4sRecoveryMDSecRwLtStLgrstOtwdInwdPos_Below160_Val/1 -> Terminator_53/1
  PA_KeSMSw4sRecoveryMDSecRwLtStLgrstOtwdInwdPos_Over180_Val/1 -> Terminator_54/1
  PA_KeSMSw4sVIPMDSecRwLtStLgrstOtwdInwdPosMax_160_Val/1 -> Terminator_55/1
  PA_KeSMSw4sVIPMDSecRwLtStLgrstOtwdInwdPosMax_165_Val/1 -> Terminator_56/1
  PA_KeSMSw4sVIPMDSecRwLtStLgrstOtwdInwdPosMax_170_Val/1 -> Terminator_57/1
  PA_KeSMSw4sVIPMDSecRwLtStLgrstOtwdInwdPosMax_175_Val/1 -> Terminator_58/1
  PA_KeSMSw4sVIPMDSecRwLtStLgrstOtwdInwdPosMax_180_Val/1 -> Terminator_59/1
  PA_KeSMSw4sVIPMDSecRwLtStLgrstOtwdInwdPosMax_Below160_Val/1 -> Terminator_60/1
  PA_KeSMSw4sVIPMDSecRwLtStLgrstOtwdInwdPosMax_Over180_Val/1 -> Terminator_61/1
  PA_KeSMSw4sVIPMDSecRwLtStLgrstOtwdInwdPosMin_160_Val/1 -> Terminator_62/1
  PA_KeSMSw4sVIPMDSecRwLtStLgrstOtwdInwdPosMin_165_Val/1 -> Terminator_63/1
  PA_KeSMSw4sVIPMDSecRwLtStLgrstOtwdInwdPosMin_170_Val/1 -> Terminator_64/1
  PA_KeSMSw4sVIPMDSecRwLtStLgrstOtwdInwdPosMin_175_Val/1 -> Terminator_65/1
  PA_KeSMSw4sVIPMDSecRwLtStLgrstOtwdInwdPosMin_180_Val/1 -> Terminator_66/1
  PA_KeSMSw4sVIPMDSecRwLtStLgrstOtwdInwdPosMin_Below160_Val/1 -> Terminator_67/1
  PA_KeSMSw4sVIPMDSecRwLtStLgrstOtwdInwdPosMin_Over180_Val/1 -> Terminator_68/1
  PA_KeSMSw4sVIPMDSecRwLtStLgrstOtwdInwdPos_160_Val/1 -> Terminator_69/1
  PA_KeSMSw4sVIPMDSecRwLtStLgrstOtwdInwdPos_165_Val/1 -> Terminator_70/1
  PA_KeSMSw4sVIPMDSecRwLtStLgrstOtwdInwdPos_170_Val/1 -> Terminator_71/1
  PA_KeSMSw4sVIPMDSecRwLtStLgrstOtwdInwdPos_175_Val/1 -> Terminator_72/1
  PA_KeSMSw4sVIPMDSecRwLtStLgrstOtwdInwdPos_180_Val/1 -> Terminator_73/1
  PA_KeSMSw4sVIPMDSecRwLtStLgrstOtwdInwdPos_Below160_Val/1 -> Terminator_74/1
  PA_KeSMSw4sVIPMDSecRwLtStLgrstOtwdInwdPos_Over180_Val/1 -> Terminator_75/1
  PA_KeSMSw6sAcsEntrySecRwLtStLgrstInwdOtwdPosMax_Val/1 -> Terminator_76/1
  PA_KeSMSw6sAcsEntrySecRwLtStLgrstInwdOtwdPosMin_Val/1 -> Terminator_77/1
  PA_KeSMSw6sAcsEntrySecRwLtStLgrstInwdOtwdPos_Val/1 -> Terminator_78/1
  PA_KeSMSw6sRecoveryMdSecRwLtStLgrstInwdOtwdPosMax_Val/1 -> Terminator_79/1
  PA_KeSMSw6sRecoveryMdSecRwLtStLgrstInwdOtwdPosMin_Val/1 -> Terminator_80/1
  PA_KeSMSw6sRecoveryMdSecRwLtStLgrstInwdOtwdPos_Val/1 -> Terminator_81/1
  PA_KeSMSwAcsEntrySecRwLtStLgrstInwdOtwdPosMax_Val/1 -> Terminator_82/1
  PA_KeSMSwAcsEntrySecRwLtStLgrstInwdOtwdPosMin_Val/1 -> Terminator_83/1
  PA_KeSMSwAcsEntrySecRwLtStLgrstInwdOtwdPos_Val/1 -> Terminator_84/1
  PA_KeSMSwRecoveryMdSecRwLtStLgrstInwdOtwdPosMax_Val/1 -> Terminator_85/1
  PA_KeSMSwRecoveryMdSecRwLtStLgrstInwdOtwdPosMin_Val/1 -> Terminator_86/1
  PA_KeSMSwRecoveryMdSecRwLtStLgrstInwdOtwdPos_Val/1 -> Terminator_87/1
  PA_KeSMSwVIPMdSecRwLtStLgrstInwdOtwdPosMax_Val/1 -> Terminator_88/1
  PA_KeSMSwVIPMdSecRwLtStLgrstInwdOtwdPosMin_Val/1 -> Terminator_89/1
  PA_KeSMSwVIPMdSecRwLtStLgrstInwdOtwdPos_Val/1 -> Terminator_90/1
  PA_KeSMSwAcsMd8SecRwLtStLgrstInwdOtwdPosMax_Val/1 -> Terminator_91/1
  PA_KeSMSwAcsMd8SecRwLtStLgrstInwdOtwdPosMin_Val/1 -> Terminator_92/1
  PA_KeSMSwAcsMd8SecRwLtStLgrstInwdOtwdPos_Val/1 -> Terminator_93/1
  PA_KeSMSw6SVIPMdSecRwLtStLgrstInwdOtwdPosMax_Val/1 -> Terminator_94/1
  PA_KeSMSw6SVIPMdSecRwLtStLgrstInwdOtwdPosMin_Val/1 -> Terminator_95/1
  PA_KeSMSw6SVIPMdSecRwLtStLgrstInwdOtwdPos_Val/1 -> Terminator_96/1

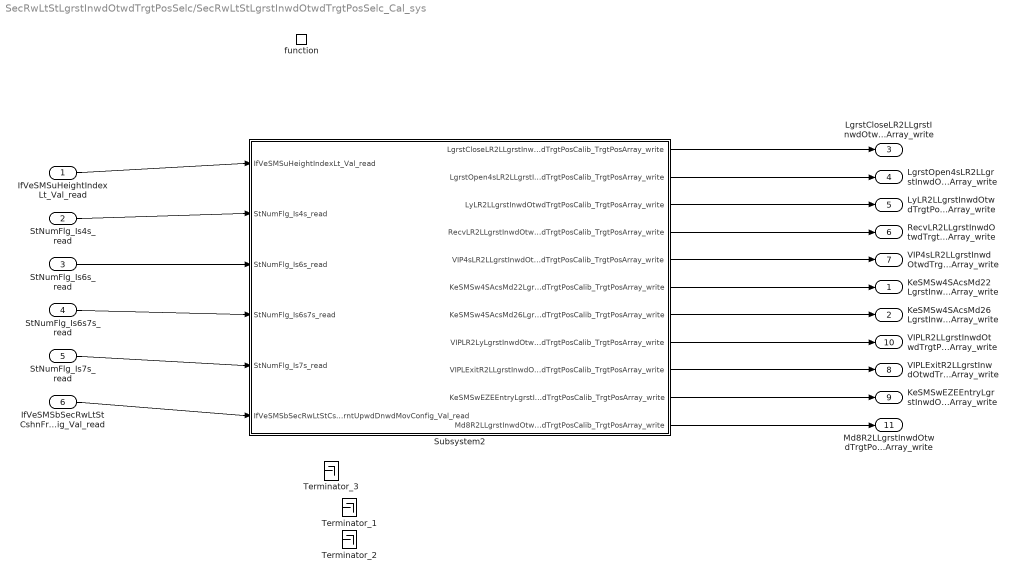
== system SecRwLtStLgrstInwdOtwdTrgtPosSelc/SecRwLtStLgrstInwdOtwdTrgtPosSelc_Cal_sys ==
  IfVeSMSuHeightIndexLt_Val_read : Inport
  StNumFlg_Is4s_read : Inport  Port=2
  StNumFlg_Is6s_read : Inport  Port=3
  StNumFlg_Is6s7s_read : Inport  Port=4
  StNumFlg_Is7s_read : Inport  Port=5
  IfVeSMSbSecRwLtStCshnFrntUpwdDnwdMovConfig_Val_read : Inport  Port=6
  function : TriggerPort  TriggerType=function-call  IsSimulinkFunction=on  FunctionName=SecRwLtStLgrstInwdOtwdTrgtPosSelc_Cal  VariantControl=(inherit)
  Subsystem2 : Subsystem
  Terminator_1 : Terminator
  Terminator_2 : Terminator
  Terminator_3 : Terminator
  KeSMSw4SAcsMd22LgrstInwdOtwdTrgtPosCalib_TrgtPosArray_write : Outport
      settings: EnsureOutportIsVirtual=on
  KeSMSw4SAcsMd26LgrstInwdOtwdTrgtPosCalib_TrgtPosArray_write : Outport  Port=2
      settings: EnsureOutportIsVirtual=on
  LgrstCloseLR2LLgrstInwdOtwdTrgtPosCalib_TrgtPosArray_write : Outport  Port=3
      settings: EnsureOutportIsVirtual=on
  LgrstOpen4sLR2LLgrstInwdOtwdTrgtPosCalib_TrgtPosArray_write : Outport  Port=4
      settings: EnsureOutportIsVirtual=on
  LyLR2LLgrstInwdOtwdTrgtPosCalib_TrgtPosArray_write : Outport  Port=5
      settings: EnsureOutportIsVirtual=on
  RecvLR2LLgrstInwdOtwdTrgtPosCalib_TrgtPosArray_write : Outport  Port=6
      settings: EnsureOutportIsVirtual=on
  VIP4sLR2LLgrstInwdOtwdTrgtPosCalib_TrgtPosArray_write : Outport  Port=7
      settings: EnsureOutportIsVirtual=on
  VIPLExitR2LLgrstInwdOtwdTrgtPosCalib_TrgtPosArray_write : Outport  Port=8
      settings: EnsureOutportIsVirtual=on
  KeSMSwEZEEntryLgrstInwdOtwdTrgtPosCalib_TrgtPosArray_write : Outport  Port=9
      settings: EnsureOutportIsVirtual=on
  VIPLR2LLgrstInwdOtwdTrgtPosCalib_TrgtPosArray_write : Outport  Port=10
      settings: EnsureOutportIsVirtual=on
  Md8R2LLgrstInwdOtwdTrgtPosCalib_TrgtPosArray_write : Outport  Port=11
      settings: EnsureOutportIsVirtual=on
  wires:
  Subsystem2/1(LgrstCloseLR2LLgrstInwdOtwdTrgtPosCalib_TrgtPosArray_write) -> LgrstCloseLR2LLgrstInwdOtwdTrgtPosCalib_TrgtPosArray_write/1
  Subsystem2/2(LgrstOpen4sLR2LLgrstInwdOtwdTrgtPosCalib_TrgtPosArray_write) -> LgrstOpen4sLR2LLgrstInwdOtwdTrgtPosCalib_TrgtPosArray_write/1
  Subsystem2/3(LyLR2LLgrstInwdOtwdTrgtPosCalib_TrgtPosArray_write) -> LyLR2LLgrstInwdOtwdTrgtPosCalib_TrgtPosArray_write/1
  Subsystem2/4(RecvLR2LLgrstInwdOtwdTrgtPosCalib_TrgtPosArray_write) -> RecvLR2LLgrstInwdOtwdTrgtPosCalib_TrgtPosArray_write/1
  Subsystem2/5(VIP4sLR2LLgrstInwdOtwdTrgtPosCalib_TrgtPosArray_write) -> VIP4sLR2LLgrstInwdOtwdTrgtPosCalib_TrgtPosArray_write/1
  Subsystem2/6(KeSMSw4SAcsMd22LgrstInwdOtwdTrgtPosCalib_TrgtPosArray_write) -> KeSMSw4SAcsMd22LgrstInwdOtwdTrgtPosCalib_TrgtPosArray_write/1
  Subsystem2/7(KeSMSw4SAcsMd26LgrstInwdOtwdTrgtPosCalib_TrgtPosArray_write) -> KeSMSw4SAcsMd26LgrstInwdOtwdTrgtPosCalib_TrgtPosArray_write/1
  IfVeSMSuHeightIndexLt_Val_read/1 -> Subsystem2/1(IfVeSMSuHeightIndexLt_Val_read)
  StNumFlg_Is4s_read/1 -> Subsystem2/2(StNumFlg_Is4s_read)
  StNumFlg_Is6s_read/1 -> Subsystem2/3(StNumFlg_Is6s_read)
  StNumFlg_Is6s7s_read/1 -> Subsystem2/4(StNumFlg_Is6s7s_read)
  StNumFlg_Is7s_read/1 -> Subsystem2/5(StNumFlg_Is7s_read)
  IfVeSMSbSecRwLtStCshnFrntUpwdDnwdMovConfig_Val_read/1 -> Subsystem2/6(IfVeSMSbSecRwLtStCshnFrntUpwdDnwdMovConfig_Val_read)
  Subsystem2/9(VIPLExitR2LLgrstInwdOtwdTrgtPosCalib_TrgtPosArray_write) -> VIPLExitR2LLgrstInwdOtwdTrgtPosCalib_TrgtPosArray_write/1
  Subsystem2/10(KeSMSwEZEEntryLgrstInwdOtwdTrgtPosCalib_TrgtPosArray_write) -> KeSMSwEZEEntryLgrstInwdOtwdTrgtPosCalib_TrgtPosArray_write/1
  Subsystem2/8(VIPLR2LyLgrstInwdOtwdTrgtPosCalib_TrgtPosArray_write) -> VIPLR2LLgrstInwdOtwdTrgtPosCalib_TrgtPosArray_write/1
  Subsystem2/11(Md8R2LLgrstInwdOtwdTrgtPosCalib_TrgtPosArray_write) -> Md8R2LLgrstInwdOtwdTrgtPosCalib_TrgtPosArray_write/1
  ? -> Terminator_1/1
  ? -> Terminator_2/1
  ? -> Terminator_3/1

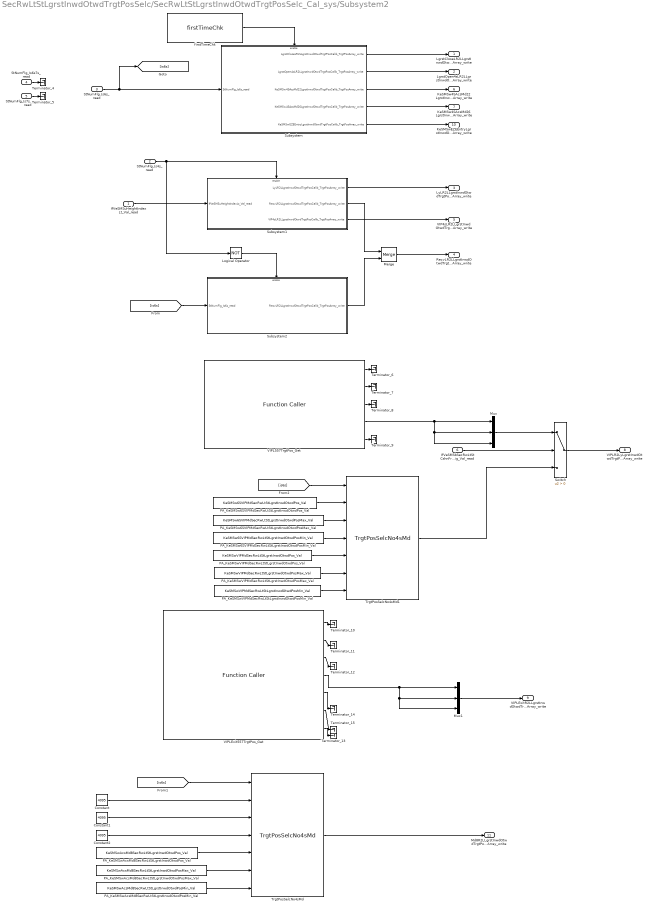
== system SecRwLtStLgrstInwdOtwdTrgtPosSelc/SecRwLtStLgrstInwdOtwdTrgtPosSelc_Cal_sys/Subsystem2 ==
  IfVeSMSuHeightIndexLt_Val_read : Inport
  StNumFlg_Is4s_read : Inport  Port=2
  StNumFlg_Is6s_read : Inport  Port=3
  StNumFlg_Is6s7s_read : Inport  Port=4
  StNumFlg_Is7s_read : Inport  Port=5
  IfVeSMSbSecRwLtStCshnFrntUpwdDnwdMovConfig_Val_read : Inport  Port=6
  Constant : Constant  Value=4095  OutDataTypeStr=uint16
  Constant1 : Constant  Value=4095  OutDataTypeStr=uint16
  Constant2 : Constant  Value=4095  OutDataTypeStr=uint16
  Logical Operator : Logic  Operator=NOT  AllPortsSameDT=off  OutDataTypeStr=boolean
  Merge : Merge
  Mux : Mux  Inputs=3
  Mux1 : Mux  Inputs=3
  PA_KeSMSw6SVIPMdSecRwLtStLgrstInwdOtwdPosMax_Val : Constant  Value=KeSMSw6SVIPMdSecRwLtStLgrstInwdOtwdPosMax_Val
  PA_KeSMSw6SVIPMdSecRwLtStLgrstInwdOtwdPosMin_Val : Constant  Value=KeSMSw6SVIPMdSecRwLtStLgrstInwdOtwdPosMin_Val
  PA_KeSMSw6SVIPMdSecRwLtStLgrstInwdOtwdPos_Val : Constant  Value=KeSMSw6SVIPMdSecRwLtStLgrstInwdOtwdPos_Val
  PA_KeSMSwAcsMd8SecRwLtStLgrstInwdOtwdPosMax_Val : Constant  Value=KeSMSwAcsMd8SecRwLtStLgrstInwdOtwdPosMax_Val
  PA_KeSMSwAcsMd8SecRwLtStLgrstInwdOtwdPosMin_Val : Constant  Value=KeSMSwAcsMd8SecRwLtStLgrstInwdOtwdPosMin_Val
  PA_KeSMSwAcsMd8SecRwLtStLgrstInwdOtwdPos_Val : Constant  Value=KeSMSwAcsMd8SecRwLtStLgrstInwdOtwdPos_Val
  PA_KeSMSwVIPMdSecRwLtStLgrstInwdOtwdPosMax_Val : Constant  Value=KeSMSwVIPMdSecRwLtStLgrstInwdOtwdPosMax_Val
  PA_KeSMSwVIPMdSecRwLtStLgrstInwdOtwdPosMin_Val : Constant  Value=KeSMSwVIPMdSecRwLtStLgrstInwdOtwdPosMin_Val
  PA_KeSMSwVIPMdSecRwLtStLgrstInwdOtwdPos_Val : Constant  Value=KeSMSwVIPMdSecRwLtStLgrstInwdOtwdPos_Val
  Subsystem : Subsystem
  Subsystem1 : Subsystem
  Subsystem2 : Subsystem
  Switch : Switch  Criteria=u2 > Threshold
  Terminator_{4..15} (12 alike) : Terminator
  TrgtPosSelcNo4sMd : TrgtPosSelcLib/TrgtPosSelcNo4sMd  SystemSampleTime=-1
  TrgtPosSelcNo4sMd1 : TrgtPosSelcLib/TrgtPosSelcNo4sMd  SystemSampleTime=-1
  VIPL557TrgtPos_Get : FunctionCaller  FunctionPrototype=[SecRwLtStBkReclnTrgtPos,SecRwLtStZeroTrgtPos,SecRwLtStLgrstUpwdDnwdTrgtPos,SecRwLtStLgrstInwdOtwdTrgtPos,SecRwLtStFwdBkwdTrgtPos] = VIPL557TrgtPos_Get()  OutputArgumentSpecifications=uint16(1), uint16(1), uint16(1), uint16(1), uint16(1)
  VIPLExit557TrgtPos_Get : FunctionCaller  FunctionPrototype=[SecRwLtStBkReclnTrgtPos,SecRwLtStZeroTrgtPos,SecRwLtStLgrstUpwdDnwdTrgtPos,SecRwLtStLgrstInwdOtwdTrgtPos,ThdRwLtStBkReclnTrgtPos,ThdRwLtStFwdBkwdTrgtPos,SecRwLtStFwdBkwdTrgtPos] = VIPLExit557TrgtPos_Get()  OutputArgumentSpecifications=uint16(1), uint16(1), uint16(1), uint16(1), uint16(1), uint16(1), uint16(1)
  firstTimeChk : TrgtPosSelcLib/firstTimeChk  SystemSampleTime=-1
  LgrstCloseLR2LLgrstInwdOtwdTrgtPosCalib_TrgtPosArray_write : Outport
      settings: EnsureOutportIsVirtual=on
  LgrstOpen4sLR2LLgrstInwdOtwdTrgtPosCalib_TrgtPosArray_write : Outport  Port=2
      settings: EnsureOutportIsVirtual=on
  LyLR2LLgrstInwdOtwdTrgtPosCalib_TrgtPosArray_write : Outport  Port=3
      settings: EnsureOutportIsVirtual=on
  RecvLR2LLgrstInwdOtwdTrgtPosCalib_TrgtPosArray_write : Outport  Port=4
      settings: EnsureOutportIsVirtual=on
  VIP4sLR2LLgrstInwdOtwdTrgtPosCalib_TrgtPosArray_write : Outport  Port=5
      settings: EnsureOutportIsVirtual=on
  KeSMSw4SAcsMd22LgrstInwdOtwdTrgtPosCalib_TrgtPosArray_write : Outport  Port=6
      settings: EnsureOutportIsVirtual=on
  KeSMSw4SAcsMd26LgrstInwdOtwdTrgtPosCalib_TrgtPosArray_write : Outport  Port=7
      settings: EnsureOutportIsVirtual=on
  VIPLR2LyLgrstInwdOtwdTrgtPosCalib_TrgtPosArray_write : Outport  Port=8
      settings: EnsureOutportIsVirtual=on
  VIPLExitR2LLgrstInwdOtwdTrgtPosCalib_TrgtPosArray_write : Outport  Port=9
      settings: EnsureOutportIsVirtual=on
  KeSMSwEZEEntryLgrstInwdOtwdTrgtPosCalib_TrgtPosArray_write : Outport  Port=10
      settings: EnsureOutportIsVirtual=on
  Md8R2LLgrstInwdOtwdTrgtPosCalib_TrgtPosArray_write : Outport  Port=11
      settings: EnsureOutportIsVirtual=on
  wires:
  StNumFlg_Is7s_read/1 -> Terminator_5/1
  Subsystem/2(LgrstOpen4sLR2LLgrstInwdOtwdTrgtPosCalib_TrgtPosArray_write) -> LgrstOpen4sLR2LLgrstInwdOtwdTrgtPosCalib_TrgtPosArray_write/1
  Subsystem1/1(LyLR2LLgrstInwdOtwdTrgtPosCalib_TrgtPosArray_write) -> LyLR2LLgrstInwdOtwdTrgtPosCalib_TrgtPosArray_write/1
  Subsystem/1(LgrstCloseLR2LLgrstInwdOtwdTrgtPosCalib_TrgtPosArray_write) -> LgrstCloseLR2LLgrstInwdOtwdTrgtPosCalib_TrgtPosArray_write/1
  StNumFlg_Is4s_read/1 -> Logical Operator/1, Subsystem1/Enable
  firstTimeChk/1 -> Subsystem/Enable
  StNumFlg_Is6s7s_read/1 -> Terminator_4/1
  Subsystem1/3(VIP4sLR2LLgrstInwdOtwdTrgtPosCalib_TrgtPosArray_write) -> VIP4sLR2LLgrstInwdOtwdTrgtPosCalib_TrgtPosArray_write/1
  IfVeSMSuHeightIndexLt_Val_read/1 -> Subsystem1/1(IfVeSMSuHeightIndexLt_Val_read)
  StNumFlg_Is6s_read/1 -> [is6s], Subsystem/1(StNumFlg_Is6s_read)
  Subsystem/4(KeSMSw4SAcsMd26LgrstInwdOtwdTrgtPosCalib_TrgtPosArray_write) -> KeSMSw4SAcsMd26LgrstInwdOtwdTrgtPosCalib_TrgtPosArray_write/1
  Subsystem/3(KeSMSw4SAcsMd22LgrstInwdOtwdTrgtPosCalib_TrgtPosArray_write) -> KeSMSw4SAcsMd22LgrstInwdOtwdTrgtPosCalib_TrgtPosArray_write/1
  Logical Operator/1 -> Subsystem2/Enable
  [is6s] -> Subsystem2/1(StNumFlg_Is6s_read)
  Subsystem2/1(RecvLR2LLgrstInwdOtwdTrgtPosCalib_TrgtPosArray_write) -> Merge/2
  Subsystem1/2(RecvLR2LLgrstInwdOtwdTrgtPosCalib_TrgtPosArray_write) -> Merge/1
  Merge/1 -> RecvLR2LLgrstInwdOtwdTrgtPosCalib_TrgtPosArray_write/1
  Switch/1 -> VIPLR2LyLgrstInwdOtwdTrgtPosCalib_TrgtPosArray_write/1
  IfVeSMSbSecRwLtStCshnFrntUpwdDnwdMovConfig_Val_read/1 -> Switch/2
  Mux/1 -> Switch/1
  VIPL557TrgtPos_Get/4 -> Mux/1, Mux/3, Mux/2
  VIPL557TrgtPos_Get/1 -> Terminator_6/1
  VIPL557TrgtPos_Get/2 -> Terminator_7/1
  VIPL557TrgtPos_Get/3 -> Terminator_8/1
  VIPL557TrgtPos_Get/5 -> Terminator_9/1
  VIPLExit557TrgtPos_Get/1 -> Terminator_10/1
  VIPLExit557TrgtPos_Get/2 -> Terminator_11/1
  VIPLExit557TrgtPos_Get/3 -> Terminator_12/1
  VIPLExit557TrgtPos_Get/5 -> Terminator_14/1
  VIPLExit557TrgtPos_Get/6 -> Terminator_15/1
  Mux1/1 -> VIPLExitR2LLgrstInwdOtwdTrgtPosCalib_TrgtPosArray_write/1
  VIPLExit557TrgtPos_Get/4 -> Mux1/2, Mux1/3, Mux1/1
  Subsystem/5(KeSMSwEZEEntryLgrstInwdOtwdTrgtPosCalib_TrgtPosArray_write) -> KeSMSwEZEEntryLgrstInwdOtwdTrgtPosCalib_TrgtPosArray_write/1
  VIPLExit557TrgtPos_Get/7 -> Terminator_13/1
  TrgtPosSelcNo4sMd/1 -> Md8R2LLgrstInwdOtwdTrgtPosCalib_TrgtPosArray_write/1
  [is6s] -> TrgtPosSelcNo4sMd/1
  PA_KeSMSwAcsMd8SecRwLtStLgrstInwdOtwdPos_Val/1 -> TrgtPosSelcNo4sMd/5
  PA_KeSMSwAcsMd8SecRwLtStLgrstInwdOtwdPosMax_Val/1 -> TrgtPosSelcNo4sMd/6
  PA_KeSMSwAcsMd8SecRwLtStLgrstInwdOtwdPosMin_Val/1 -> TrgtPosSelcNo4sMd/7
  Constant/1 -> TrgtPosSelcNo4sMd/2
  Constant1/1 -> TrgtPosSelcNo4sMd/3
  Constant2/1 -> TrgtPosSelcNo4sMd/4
  TrgtPosSelcNo4sMd1/1 -> Switch/3
  [is6s] -> TrgtPosSelcNo4sMd1/1
  PA_KeSMSw6SVIPMdSecRwLtStLgrstInwdOtwdPosMax_Val/1 -> TrgtPosSelcNo4sMd1/3
  PA_KeSMSw6SVIPMdSecRwLtStLgrstInwdOtwdPosMin_Val/1 -> TrgtPosSelcNo4sMd1/4
  PA_KeSMSw6SVIPMdSecRwLtStLgrstInwdOtwdPos_Val/1 -> TrgtPosSelcNo4sMd1/2
  PA_KeSMSwVIPMdSecRwLtStLgrstInwdOtwdPosMax_Val/1 -> TrgtPosSelcNo4sMd1/6
  PA_KeSMSwVIPMdSecRwLtStLgrstInwdOtwdPos_Val/1 -> TrgtPosSelcNo4sMd1/5
  PA_KeSMSwVIPMdSecRwLtStLgrstInwdOtwdPosMin_Val/1 -> TrgtPosSelcNo4sMd1/7

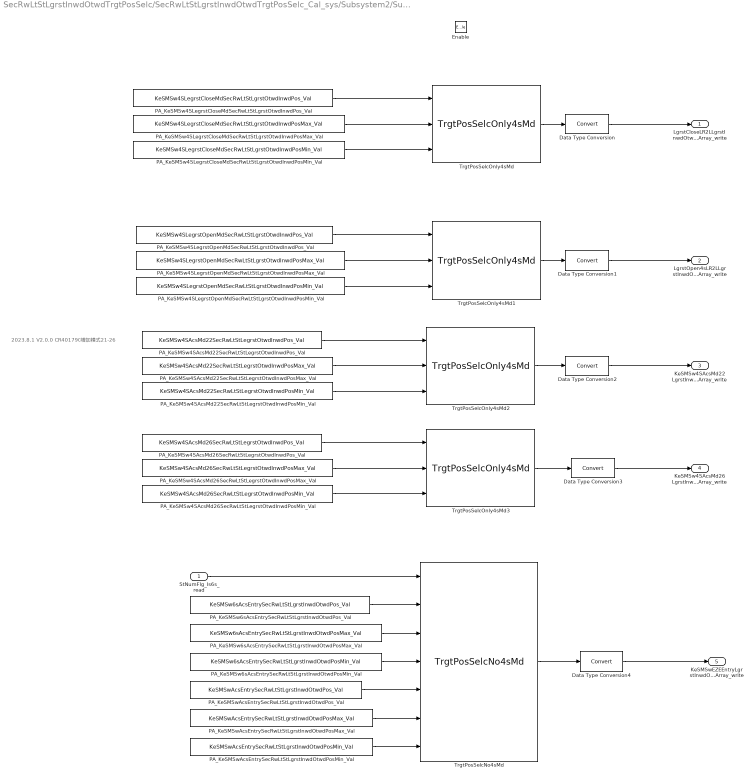
== system SecRwLtStLgrstInwdOtwdTrgtPosSelc/SecRwLtStLgrstInwdOtwdTrgtPosSelc_Cal_sys/Subsystem2/Subsystem ==
  note: 2023.8.1 V2.0.0 CR401790 增加模式21-26
  StNumFlg_Is6s_read : Inport
  Enable : EnablePort
  Data Type Conversion{,1..4} (5 alike) : DataTypeConversion
  PA_KeSMSw4SAcsMd22SecRwLtStLegrstOtwdInwdPosMax_Val : Constant  Value=KeSMSw4SAcsMd22SecRwLtStLegrstOtwdInwdPosMax_Val
  PA_KeSMSw4SAcsMd22SecRwLtStLegrstOtwdInwdPosMin_Val : Constant  Value=KeSMSw4SAcsMd22SecRwLtStLegrstOtwdInwdPosMin_Val
  PA_KeSMSw4SAcsMd22SecRwLtStLegrstOtwdInwdPos_Val : Constant  Value=KeSMSw4SAcsMd22SecRwLtStLegrstOtwdInwdPos_Val
  PA_KeSMSw4SAcsMd26SecRwLtStLegrstOtwdInwdPosMax_Val : Constant  Value=KeSMSw4SAcsMd26SecRwLtStLegrstOtwdInwdPosMax_Val
  PA_KeSMSw4SAcsMd26SecRwLtStLegrstOtwdInwdPosMin_Val : Constant  Value=KeSMSw4SAcsMd26SecRwLtStLegrstOtwdInwdPosMin_Val
  PA_KeSMSw4SAcsMd26SecRwLtStLegrstOtwdInwdPos_Val : Constant  Value=KeSMSw4SAcsMd26SecRwLtStLegrstOtwdInwdPos_Val
  PA_KeSMSw4SLegrstCloseMdSecRwLtStLgrstOtwdInwdPosMax_Val : Constant  Value=KeSMSw4SLegrstCloseMdSecRwLtStLgrstOtwdInwdPosMax_Val
  PA_KeSMSw4SLegrstCloseMdSecRwLtStLgrstOtwdInwdPosMin_Val : Constant  Value=KeSMSw4SLegrstCloseMdSecRwLtStLgrstOtwdInwdPosMin_Val
  PA_KeSMSw4SLegrstCloseMdSecRwLtStLgrstOtwdInwdPos_Val : Constant  Value=KeSMSw4SLegrstCloseMdSecRwLtStLgrstOtwdInwdPos_Val
  PA_KeSMSw4SLegrstOpenMdSecRwLtStLgrstOtwdInwdPosMax_Val : Constant  Value=KeSMSw4SLegrstOpenMdSecRwLtStLgrstOtwdInwdPosMax_Val
  PA_KeSMSw4SLegrstOpenMdSecRwLtStLgrstOtwdInwdPosMin_Val : Constant  Value=KeSMSw4SLegrstOpenMdSecRwLtStLgrstOtwdInwdPosMin_Val
  PA_KeSMSw4SLegrstOpenMdSecRwLtStLgrstOtwdInwdPos_Val : Constant  Value=KeSMSw4SLegrstOpenMdSecRwLtStLgrstOtwdInwdPos_Val
  PA_KeSMSw6sAcsEntrySecRwLtStLgrstInwdOtwdPosMax_Val : Constant  Value=KeSMSw6sAcsEntrySecRwLtStLgrstInwdOtwdPosMax_Val
  PA_KeSMSw6sAcsEntrySecRwLtStLgrstInwdOtwdPosMin_Val : Constant  Value=KeSMSw6sAcsEntrySecRwLtStLgrstInwdOtwdPosMin_Val
  PA_KeSMSw6sAcsEntrySecRwLtStLgrstInwdOtwdPos_Val : Constant  Value=KeSMSw6sAcsEntrySecRwLtStLgrstInwdOtwdPos_Val
  PA_KeSMSwAcsEntrySecRwLtStLgrstInwdOtwdPosMax_Val : Constant  Value=KeSMSwAcsEntrySecRwLtStLgrstInwdOtwdPosMax_Val
  PA_KeSMSwAcsEntrySecRwLtStLgrstInwdOtwdPosMin_Val : Constant  Value=KeSMSwAcsEntrySecRwLtStLgrstInwdOtwdPosMin_Val
  PA_KeSMSwAcsEntrySecRwLtStLgrstInwdOtwdPos_Val : Constant  Value=KeSMSwAcsEntrySecRwLtStLgrstInwdOtwdPos_Val
  TrgtPosSelcNo4sMd : TrgtPosSelcLib/TrgtPosSelcNo4sMd  SystemSampleTime=-1
  TrgtPosSelcOnly4sMd{,1..3} (4 alike) : TrgtPosSelcLib/TrgtPosSelcOnly4sMd  SystemSampleTime=-1
  LgrstCloseLR2LLgrstInwdOtwdTrgtPosCalib_TrgtPosArray_write : Outport
  LgrstOpen4sLR2LLgrstInwdOtwdTrgtPosCalib_TrgtPosArray_write : Outport  Port=2
  KeSMSw4SAcsMd22LgrstInwdOtwdTrgtPosCalib_TrgtPosArray_write : Outport  Port=3
      settings: EnsureOutportIsVirtual=on
  KeSMSw4SAcsMd26LgrstInwdOtwdTrgtPosCalib_TrgtPosArray_write : Outport  Port=4
      settings: EnsureOutportIsVirtual=on
  KeSMSwEZEEntryLgrstInwdOtwdTrgtPosCalib_TrgtPosArray_write : Outport  Port=5
      settings: EnsureOutportIsVirtual=on
  wires:
  PA_KeSMSw4SLegrstCloseMdSecRwLtStLgrstOtwdInwdPos_Val/1 -> TrgtPosSelcOnly4sMd/1
  TrgtPosSelcOnly4sMd1/1 -> Data Type Conversion1/1
  TrgtPosSelcOnly4sMd/1 -> Data Type Conversion/1
  PA_KeSMSw4SLegrstOpenMdSecRwLtStLgrstOtwdInwdPosMin_Val/1 -> TrgtPosSelcOnly4sMd1/3
  PA_KeSMSw4SLegrstOpenMdSecRwLtStLgrstOtwdInwdPosMax_Val/1 -> TrgtPosSelcOnly4sMd1/2
  PA_KeSMSw4SLegrstCloseMdSecRwLtStLgrstOtwdInwdPosMin_Val/1 -> TrgtPosSelcOnly4sMd/3
  PA_KeSMSw4SLegrstOpenMdSecRwLtStLgrstOtwdInwdPos_Val/1 -> TrgtPosSelcOnly4sMd1/1
  PA_KeSMSw4SLegrstCloseMdSecRwLtStLgrstOtwdInwdPosMax_Val/1 -> TrgtPosSelcOnly4sMd/2
  TrgtPosSelcOnly4sMd2/1 -> Data Type Conversion2/1
  TrgtPosSelcOnly4sMd3/1 -> Data Type Conversion3/1
  PA_KeSMSw4SAcsMd22SecRwLtStLegrstOtwdInwdPosMax_Val/1 -> TrgtPosSelcOnly4sMd2/2
  PA_KeSMSw4SAcsMd22SecRwLtStLegrstOtwdInwdPosMin_Val/1 -> TrgtPosSelcOnly4sMd2/3
  PA_KeSMSw4SAcsMd22SecRwLtStLegrstOtwdInwdPos_Val/1 -> TrgtPosSelcOnly4sMd2/1
  PA_KeSMSw4SAcsMd26SecRwLtStLegrstOtwdInwdPosMax_Val/1 -> TrgtPosSelcOnly4sMd3/2
  PA_KeSMSw4SAcsMd26SecRwLtStLegrstOtwdInwdPosMin_Val/1 -> TrgtPosSelcOnly4sMd3/3
  PA_KeSMSw4SAcsMd26SecRwLtStLegrstOtwdInwdPos_Val/1 -> TrgtPosSelcOnly4sMd3/1
  Data Type Conversion/1 -> LgrstCloseLR2LLgrstInwdOtwdTrgtPosCalib_TrgtPosArray_write/1
  Data Type Conversion1/1 -> LgrstOpen4sLR2LLgrstInwdOtwdTrgtPosCalib_TrgtPosArray_write/1
  Data Type Conversion2/1 -> KeSMSw4SAcsMd22LgrstInwdOtwdTrgtPosCalib_TrgtPosArray_write/1
  Data Type Conversion3/1 -> KeSMSw4SAcsMd26LgrstInwdOtwdTrgtPosCalib_TrgtPosArray_write/1
  Data Type Conversion4/1 -> KeSMSwEZEEntryLgrstInwdOtwdTrgtPosCalib_TrgtPosArray_write/1
  TrgtPosSelcNo4sMd/1 -> Data Type Conversion4/1
  StNumFlg_Is6s_read/1 -> TrgtPosSelcNo4sMd/1
  PA_KeSMSw6sAcsEntrySecRwLtStLgrstInwdOtwdPos_Val/1 -> TrgtPosSelcNo4sMd/2
  PA_KeSMSw6sAcsEntrySecRwLtStLgrstInwdOtwdPosMax_Val/1 -> TrgtPosSelcNo4sMd/3
  PA_KeSMSw6sAcsEntrySecRwLtStLgrstInwdOtwdPosMin_Val/1 -> TrgtPosSelcNo4sMd/4
  PA_KeSMSwAcsEntrySecRwLtStLgrstInwdOtwdPos_Val/1 -> TrgtPosSelcNo4sMd/5
  PA_KeSMSwAcsEntrySecRwLtStLgrstInwdOtwdPosMax_Val/1 -> TrgtPosSelcNo4sMd/6
  PA_KeSMSwAcsEntrySecRwLtStLgrstInwdOtwdPosMin_Val/1 -> TrgtPosSelcNo4sMd/7
